simulink model "simLink_linefollower"  (R2022b)
settings: Solver=FixedStepAuto  StartTime=0.0  StopTime=10  FixedStep=0.1  RelTol=1e-3
values from neighbouring files (symbols this model uses):
  length_body = pixel_body/pixel_conversion    (= 80)    [startSim.m]
  length_close_sensor = pixel_body/pixel_conversion    (= 80)    [startSim.m]
  map = zeros(map_size_x, map_size_y)    [generate_map.m]    (also in startSim.m = imcomplement(map))
  pixel_sensor = 3    [startSim.m]
  Position_noise = 0    [startSim.m]
  reading_noise = 0    [startSim.m]
  spacing = 2/pixel_conversion    (= 20)    [startSim.m]
  velocity_left = 80    [startSim.m]
  velocity_right = 80    [startSim.m]
undefined symbols (not defined in the file or in its folder): offset_x, offset_y
libraries: simulink x28, slpidlib x1, robotmobilelib x1
(part 2 of 2)

== matlab function simLink_linefollower/Calculate sensor_close values/MATLAB Function ==
  data: coord input; sensor_values output; img input; offset_x input; offset_y input; pixel input; pos output
function [sensor_values, pos] = fcn(coord, img, offset_x,offset_y, pixel)

sensor_values = zeros(7,1);
sensor_ones = ones(pixel*2+1,pixel*2+1);
pos = zeros(14,1);


x1 = round(coord(1) + offset_x);
y1 = round(coord(2) + offset_y);
x2 = round(coord(3) + offset_x);
y2 = round(coord(4) + offset_y);
x3 = round(coord(5) + offset_x);
y3 = round(coord(6) + offset_y);
x4 = round(coord(7) + offset_x);
y4 = round(coord(8) + offset_y);
x5 = round(coord(9) + offset_x);
y5 = round(coord(10) + offset_y);
x6 = round(coord(11) + offset_x);
y6 = round(coord(12) + offset_y);
x7 = round(coord(13) + offset_x);
y7 = round(coord(14) + offset_y);

sens1 = img(y1 - pixel:y1 + pixel, x1 - pixel:x1 + pixel);
sens2 = img(y2 - pixel:y2 + pixel, x2 - pixel:x2 + pixel);
sens3 = img(y3 - pixel:y3 + pixel, x3 - pixel:x3 + pixel);
sens4 = img(y4 - pixel:y4 + pixel, x4 - pixel:x4 + pixel);
sens5 = img(y5 - pixel:y5 + pixel, x5 - pixel:x5 + pixel);
sens6 = img(y6 - pixel:y6 + pixel, x6 - pixel:x6 + pixel);
sens7 = img(y7 - pixel:y7 + pixel, x7 - pixel:x7 + pixel);

sensor_values(1) = sum(dot(sens1, sensor_ones),2);
sensor_values(2) = sum(dot(sens2, sensor_ones),2);
sensor_values(3) = sum(dot(sens3, sensor_ones),2);
sensor_values(4) = sum(dot(sens4, sensor_ones),2);
sensor_values(5) = sum(dot(sens5, sensor_ones),2);
sensor_values(6) = sum(dot(sens6, sensor_ones),2);
sensor_values(7) = sum(dot(sens7, sensor_ones),2);

pos(1) = x1;
pos(2) = y1;
pos(3) = x2;
pos(4) = y2;
pos(5) = x3;
pos(6) = y3;
pos(7) = x4;
pos(8) = y4;
pos(9) = x5;
pos(10) = y5;
pos(11) = x6;
pos(12) = y6;
pos(13) = x7;
pos(14) = y7;

== matlab function simLink_linefollower/Calculate sensor values/MATLAB Function ==
  data: coord input; sensor_values output; img input; offset_x input; offset_y input; pixel input; pos output
function [sensor_values, pos] = fcn(coord, img, offset_x,offset_y, pixel)

sensor_values = zeros(7,1);
sensor_ones = ones(pixel*2+1,pixel*2+1);
pos = zeros(14,1);


x1 = round(coord(1) + offset_x);
y1 = round(coord(2) + offset_y);
x2 = round(coord(3) + offset_x);
y2 = round(coord(4) + offset_y);
x3 = round(coord(5) + offset_x);
y3 = round(coord(6) + offset_y);
x4 = round(coord(7) + offset_x);
y4 = round(coord(8) + offset_y);
x5 = round(coord(9) + offset_x);
y5 = round(coord(10) + offset_y);
x6 = round(coord(11) + offset_x);
y6 = round(coord(12) + offset_y);
x7 = round(coord(13) + offset_x);
y7 = round(coord(14) + offset_y);

sens1 = img(y1 - pixel:y1 + pixel, x1 - pixel:x1 + pixel);
sens2 = img(y2 - pixel:y2 + pixel, x2 - pixel:x2 + pixel);
sens3 = img(y3 - pixel:y3 + pixel, x3 - pixel:x3 + pixel);
sens4 = img(y4 - pixel:y4 + pixel, x4 - pixel:x4 + pixel);
sens5 = img(y5 - pixel:y5 + pixel, x5 - pixel:x5 + pixel);
sens6 = img(y6 - pixel:y6 + pixel, x6 - pixel:x6 + pixel);
sens7 = img(y7 - pixel:y7 + pixel, x7 - pixel:x7 + pixel);

sensor_values(1) = sum(dot(sens1, sensor_ones),2);
sensor_values(2) = sum(dot(sens2, sensor_ones),2);
sensor_values(3) = sum(dot(sens3, sensor_ones),2);
sensor_values(4) = sum(dot(sens4, sensor_ones),2);
sensor_values(5) = sum(dot(sens5, sensor_ones),2);
sensor_values(6) = sum(dot(sens6, sensor_ones),2);
sensor_values(7) = sum(dot(sens7, sensor_ones),2);

pos(1) = x1;
pos(2) = y1;
pos(3) = x2;
pos(4) = y2;
pos(5) = x3;
pos(6) = y3;
pos(7) = x4;
pos(8) = y4;
pos(9) = x5;
pos(10) = y5;
pos(11) = x6;
pos(12) = y6;
pos(13) = x7;
pos(14) = y7;
